simulink model "OMEGA"  (R2024a)
settings: Solver=VariableStepAuto  StartTime=0.0  StopTime=10.0  RelTol=1e-3
settings Model: Creator=emanuele  LastModifiedBy=emanuele

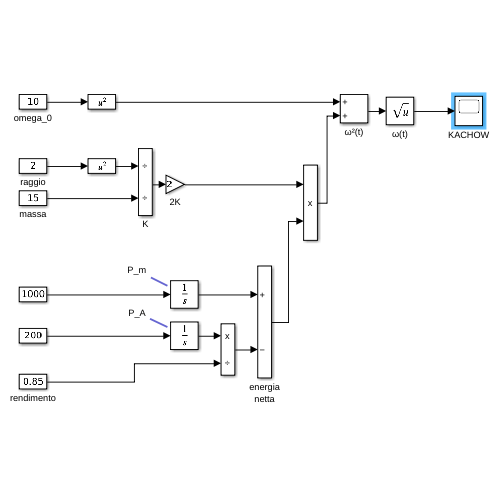
[thumbnail: Simulink's stored preview of the top-level diagram]
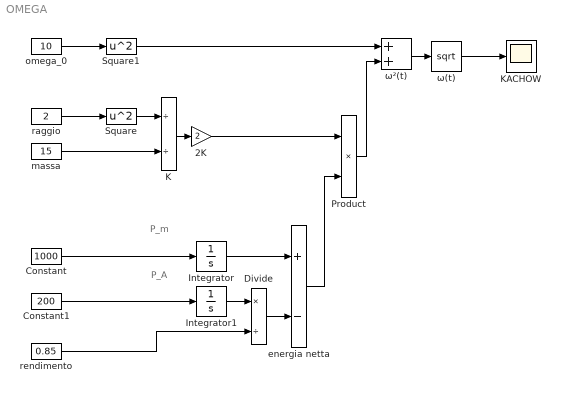
== system OMEGA ==
  note: P_m
  note: P_A
  2K : Gain  Gain=2
  Constant : Constant  Value=1000
  Constant1 : Constant  Value=200
  Divide : Product  Inputs=*/
  Integrator : Integrator
  Integrator1 : Integrator
  K : Product  Inputs=//
  KACHOW : Scope
  Product : Product
  Square : Math  Operator=square
  Square1 : Math  Operator=square
  energia netta : Sum  Inputs=+-
  massa : Constant  Value=15
  omega_0 : Constant  Value=10
  raggio : Constant  Value=2
  rendimento : Constant  Value=0.85
  ω(t) : Sqrt
  ω²(t) : Sum
  wires:
  massa/1 -> K/2
  raggio/1 -> Square/1
  Square/1 -> K/1
  K/1 -> 2K/1
  omega_0/1 -> Square1/1
  Square1/1 -> ω²(t)/1
  Product/1 -> ω²(t)/2
  2K/1 -> Product/1
  energia netta/1 -> Product/2
  Integrator/1 -> energia netta/1
  Divide/1 -> energia netta/2
  Integrator1/1 -> Divide/1
  rendimento/1 -> Divide/2
  ω²(t)/1 -> ω(t)/1
  Constant/1 -> Integrator/1
  Constant1/1 -> Integrator1/1
  ω(t)/1 -> KACHOW/1
